simulink library "mode_selection"  (R2016b)
settings: Solver=VariableStepAuto  StartTime=0.0  StopTime=10.0  RelTol=1e-3
settings Model: Creator=taylorreynolds  LastModifiedBy=Taylor

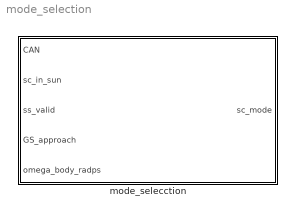
== system mode_selection ==
  mode_selecction : Subsystem

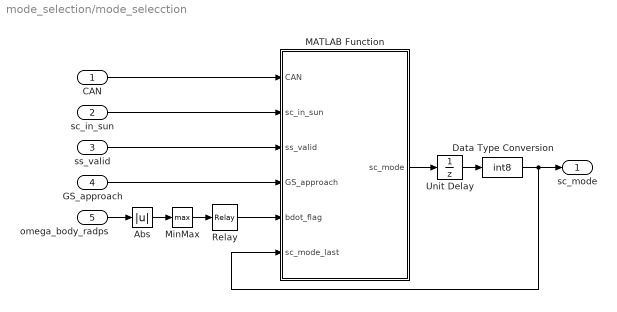
== system mode_selection/mode_selecction ==
  CAN : Inport
  sc_in_sun : Inport  Port=2
  ss_valid : Inport  Port=3
  GS_approach : Inport  Port=4
  omega_body_radps : Inport  Port=5
  Abs : Abs
  Data Type Conversion : DataTypeConversion  OutDataTypeStr=int8  RndMeth=Nearest
  MATLAB Function : MATLAB Function  TreatAsAtomicUnit=on
  MinMax : MinMax  Function=max
  Relay : Relay  OnSwitchValue=fsw_params.bus.omega_radps_thresh.max  OffSwitchValue=fsw_params.bus.omega_radps_thresh.min
  Unit Delay : UnitDelay  InitialCondition=1  SampleTime=-1
  sc_mode : Outport
  wires:
  GS_approach/1 -> MATLAB Function/4(GS_approach)
  CAN/1 -> MATLAB Function/1(CAN)
  sc_in_sun/1 -> MATLAB Function/2(sc_in_sun)
  omega_body_radps/1 -> Abs/1
  MATLAB Function/1(sc_mode) -> Unit Delay/1
  Unit Delay/1 -> Data Type Conversion/1
  Abs/1 -> MinMax/1
  MinMax/1 -> Relay/1
  Relay/1 -> MATLAB Function/5(bdot_flag)
  Data Type Conversion/1 -> sc_mode/1, MATLAB Function/6(sc_mode_last)
  ss_valid/1 -> MATLAB Function/3(ss_valid)

== matlab function mode_selection/mode_selecction/MATLAB Function ==
  data: CAN input int8; sc_in_sun input; ss_valid input; GS_approach input; bdot_flag input; sc_mode output int8; sc_mode_last input
 function sc_mode = adcs_mode_logic(CAN,sc_in_sun,ss_valid,GS_approach,bdot_flag,sc_mode_last)
% ----------------------------------------------------------------------- %
% Main FSW Mode Selector
%   UW HuskySat-1, ADCS Team
%   Last Updated: T. Reynolds 2.15.18
%
% Chooses control mode based on sensor and actuator data.
%   mode_logic.bdot             = 1;
%   mode_logic.seek_sun         = 2;
%   mode_logic.point            = 3;
%       point.velocity          = 31;
%       point.ground            = 32;
%       point.MPC               = 33;
%   mode_logic.low_power        = 4;
%
% ----- INPUTS -----
%
% CAN - Data coming over the CAN bus. Type: 6x1 double. Parsed according to:
%
%   CAN(1) == Override the autonomous mode selection and command the mode
%               corresponding to this number. Set to 0 if the autonomous 
%               selection is to go ahead.
%   CAN(2) == Reboot just occured OR we just exited a detumble. Value: BOOL. 
%               we will sit in this mode until either pointing takes over
%               or body rates rise again.
%   CAN(3) == Go ahead for the pointing mode. Value: BOOL. One means the s/c
%               is go for pointing of any kind.
%   CAN(4) == Go ahead for COM2 and GS pointing. Value: BOOL. One means that
%               the COM2 system will be booted on the next flyover.
%   CAN(5) == PPT On. Value: BOOL. Zero implies PPT is off and will not fire
%               on the next sync cycle.
%
% sc_in_sun: - Tells us if the s/c is in eclipse. Type: 1x1 boolean.
%
% ss_valid: - Valid bit from the sun sensor indicating whether or not the
% sun is in our FoV. Type: 1x1 boolean.
%
% GS_appraoch: - Tells us if the ground station is approaching based on
%                   reorientation criteria. Type: 1x1 boolean.
%
% bdot_flag: - Output from the relay block. Goes high when thresh_max is
% hit, and does not go low until thresh_min is hit (hysteresis).
%
% desat_flag: - Same as bdot_flag but with reaction wheel RPM thresholds.
%
% sc_mode_old - Previous spacecraft state, used to test exit conditions for
%                   each mode.
%
%
% ----- OUTPUTS -----
%
% sc_mode - Spacecraft state determined. Type: int8.
%
% #codegen
% ----------------------------------------------------------------------- %

% Default to last known condition and no experimental control
sc_mode     = sc_mode_last;

if( CAN(1) == 0 )
    
    % Check for bdot condition
    if( bdot_flag == 1 )
        sc_mode     = int8(1.0);
        % If Bdot is triggered, return immediately since control has high 
        % priority and control will be handed off.
        return;
    end
    
    % Bdot flag will go low once omega_radps drops below the lower
    % threshold. Accounted for in the relay block.
        
    % Check for low power condition or recent boot up
    if( CAN(2) == 1 || (sc_mode == 1 && bdot_flag == 0) )
        % If reboot/bdot just occured and we are not tumbling, enter low
        % power/estimate mode.
        sc_mode     = int8(4.0);
    end
        
    % Check if we have the sun in our FoV. If not, enter reorientation 
    % mode to acquire sun. This has high priority if we are not tumbling.
    if( sc_in_sun && (~ss_valid) )
        sc_mode     = int8(2.0);
        return;
    end
    
    % If all cases upstream have been passed, then enter pointing mode if
    % allowed to do so. Check for pointing condition from CAN
    if( CAN(3) == 1 )
        % Default to velocity pointing mode
        sc_mode     = int8(31.0);
        
        % Check to see if entering GS range, not in eclipse and
        % COM2 system will be activated.
        if( GS_approach && sc_in_sun && (CAN(4)==1) )
            sc_mode  = int8(32.0);
        end
                
    end 
    
% If signal received to override the autonomous mode selection, set mode 
% based on CAN(1) value.
elseif( CAN(1) ~= 0 )
    
    sc_mode = CAN(1);
    
end
